simulink model "Astatic_Polynomial"  (R2021a)
settings: Solver=FixedStepAuto  StartTime=0.0  StopTime=STime  FixedStep=1e-3  RelTol=1e-3
undefined symbols (not defined in the file): C, C_polya, J, Kp, Mc, r0a, R_polya, Ra, Ta, Tp, TPert
settings Model: Creator=akangmufti  LastModifiedBy=akangmufti

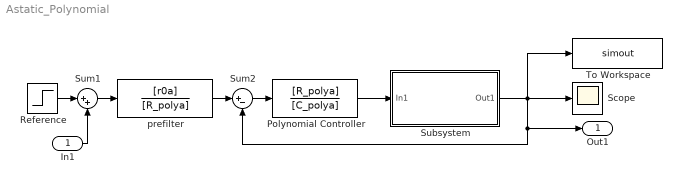
== system Astatic_Polynomial ==
  In1 : Inport
  Polynomial Controller : TransferFcn  Numerator=[R_polya]  Denominator=[C_polya]
  Reference : Step  Time=1e-3  SampleTime=0
  Scope : Scope
  Subsystem : Subsystem
  Sum1 : Sum  Inputs=|++
  Sum2 : Sum  Inputs=|+-
  To Workspace : ToWorkspace  VariableName=simout  SampleTime=-1
  prefilter : TransferFcn  Numerator=[r0a]  Denominator=[R_polya]
  Out1 : Outport
  wires:
  Sum2/1 -> Polynomial Controller/1
  Reference/1 -> Sum1/1
  Sum1/1 -> prefilter/1
  In1/1 -> Sum1/2
  Subsystem/1(Out1) -> Scope/1, To Workspace/1, Sum2/2, Out1/1
  prefilter/1 -> Sum2/1
  Polynomial Controller/1 -> Subsystem/1(In1)

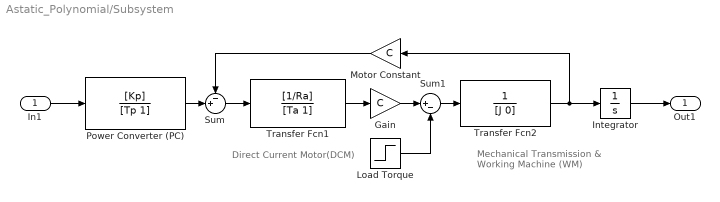
== system Astatic_Polynomial/Subsystem ==
  note: Direct Current Motor(DCM)
  note: Mechanical Transmission &
      | Working Machine (WM)
  In1 : Inport
  Gain : Gain  Gain=C
  Integrator : Integrator  ContinuousStateAttributes='AngularPosition'
  Load Torque : Step  Time=TPert  After=Mc  SampleTime=0
  Motor Constant : Gain  Gain=C
  Power Converter (PC) : TransferFcn  Numerator=[Kp]  Denominator=[Tp 1]
  Sum : Sum  Inputs=-+|
  Sum1 : Sum  Inputs=|+-
  Transfer Fcn1 : TransferFcn  Numerator=[1/Ra]  Denominator=[Ta 1]  ContinuousStateAttributes='Current'
  Transfer Fcn2 : TransferFcn  Denominator=[J 0]  ContinuousStateAttributes='Omega'
  Out1 : Outport
  wires:
  Transfer Fcn2/1 -> Integrator/1, Motor Constant/1
  Power Converter (PC)/1 -> Sum/2
  Gain/1 -> Sum1/1
  Sum1/1 -> Transfer Fcn2/1
  Sum/1 -> Transfer Fcn1/1
  Transfer Fcn1/1 -> Gain/1
  Motor Constant/1 -> Sum/1
  In1/1 -> Power Converter (PC)/1
  Load Torque/1 -> Sum1/2
  Integrator/1 -> Out1/1
